simulink library "tqr"  (R2021b)
settings: Solver=VariableStepAuto  StartTime=0.0  StopTime=10.0  RelTol=1e-3
undefined symbols (not defined in the file or in its folder): ATQR_AltRDCActiveFEDUInc_X_pct, ATQR_AltRDCActiveFEDUInc_Y_enum, ATQR_AltRDCActiveFEDUTs_X_pct, ATQR_AltRDCActiveFEDUTs_Y_enum, ATQR_AltRDCActiveREDUInc_X_pct, ATQR_AltRDCActiveREDUInc_Y_enum, ATQR_AltRDCActiveREDUTs_X_pct, ATQR_AltRDCActiveREDUTs_Y_enum, ATQR_CreepFEDUTqIncSR_X_rpm, ATQR_CreepFEDUTqIncSR_Y_Nm, ATQR_CreepFEDUTs_X_rpm, ATQR_CreepFEDUTs_Y_Nm, ATQR_EcoTqFrIncGain_X_Nm, ATQR_EcoTqFrIncGain_Y_pct, ATQR_EcoTqRrIncGain_X_Nm, ATQR_EcoTqRrIncGain_Y_pct, ATQR_EL1FEDUTqDecSR_Y_Nm, ATQR_EL1FEDUTqIncSR_X_rpm, ATQR_EL1FEDUTqIncSR_Y_pct, ATQR_EL1FEDUTs_X_rpm, ATQR_EL1FEDUTs_Y_Nm, ATQR_EL1REDUTqDecSR_Y_Nm, ATQR_EL1REDUTs_Y_Nm, ATQR_FEDUEL1RegenTs_X_rpm, ATQR_FEDUTIPOutTs_X_rpm, ATQR_FrNegRateLimitIncN_X_rpm, ATQR_FrNegRateLimitIncN_Y_Nm, ATQR_FrPosRateLimitIncN_X_rpm, ATQR_FrPosRateLimitIncN_Y_Nm, ATQR_FShaftSpdTqLimCoe_X_rpm, ATQR_FTimerTqLimCoe_X_s, ATQR_FTqZeroTransUpBoundN_X_rpm, ATQR_NL1FEDUTqDecSR_Y_Nm, ATQR_NL1FEDUTqIncSR_X_rpm, ATQR_NL1FEDUTqIncSR_Y_pct, ATQR_NL1FEDUTs_X_rpm, ATQR_NL1FEDUTs_Y_Nm, ATQR_NL1REDUTqDecSR_Y_Nm, ATQR_NL1REDUTs_Y_Nm, ATQR_NormalTqFrIncGain_X_Nm, ATQR_NormalTqFrIncGain_Y_pct, ATQR_NormalTqRrIncGain_X_Nm, ATQR_NormalTqRrIncGain_Y_pct, ATQR_RrNegRateLimitIncN_X_rpm, ATQR_RrNegRateLimitIncN_Y_Nm, ATQR_RrPosRateLimitIncN_X_rpm, ATQR_RrPosRateLimitIncN_Y_Nm, ATQR_RShaftSpdTqLimCoe_X_rpm, ATQR_RTimerTqLimCoe_X_s, ATQR_SL1FEDUTqDecSR_Y_Nm, ATQR_SL1FEDUTqIncSR_X_rpm, ATQR_SL1FEDUTqIncSR_Y_pct, ATQR_SL1FEDUTs_X_rpm, ATQR_SL1FEDUTs_Y_Nm, ATQR_SL1REDUTqDecSR_Y_Nm, ATQR_SL1REDUTs_Y_Nm, ATQR_SportTqFrIncGain_X_Nm, ATQR_SportTqFrIncGain_Y_pct, ATQR_SportTqRrIncGain_X_Nm, ATQR_SportTqRrIncGain_Y_pct ... (+287)
libraries: hcu_lib x19, simulink x17, $bdroot x3
(part 2 of 10)

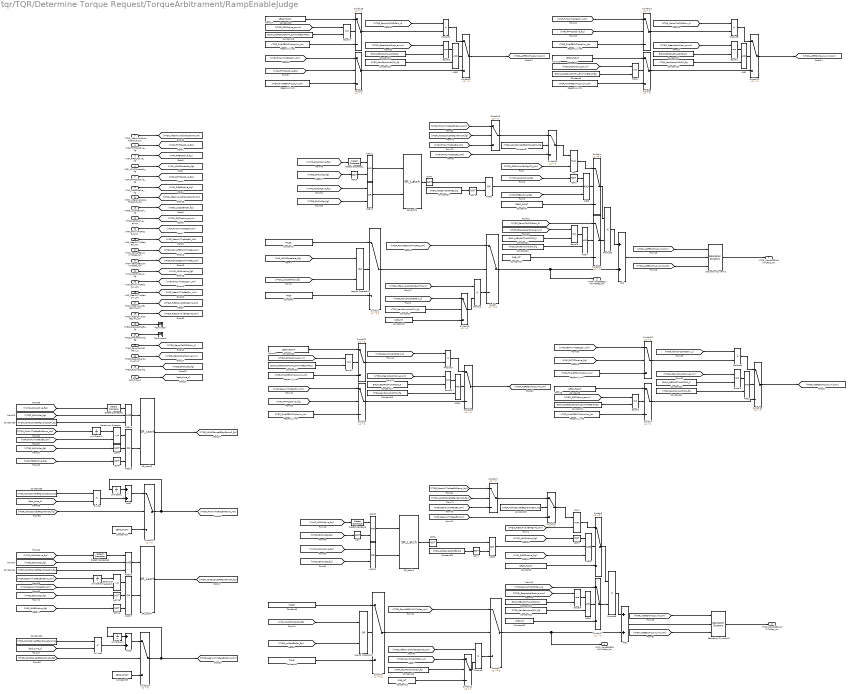
== system tqr/TQR/Determine Torque Request/TorqueArbitrament/RampEnableJudge ==
  VTQD_AfterAvailableTqDemFr_Nm : Inport
  VINP_FrPTCSActive_flg : Inport  Port=2
  VINP_FrRBCActive_flg : Inport  Port=3
  VINP_ADASForceIdle_flg : Inport  Port=4
  VTQR_RampFEDUWhlTqReq_Nm : Inport  Port=5
  VTQD_AfterAvailableTqDemRr_Nm : Inport  Port=6
  VINP_RrPTCSActive_flg : Inport  Port=7
  VINP_RrRBCActive_flg : Inport  Port=8
  VTQR_RampREDUWhlTqReq_Nm : Inport  Port=9
  VTQD_LoSpdBrkCtrl_flg : Inport  Port=10
  VTQD_RDCActive_enum : Inport  Port=11
  VINP_FrntAxlTrqReqBrk_Nm : Inport  Port=12
  VINP_RearAxlTrqReqBrk_Nm : Inport  Port=13
  VVMC_ADASActive_flg : Inport  Port=14
  VINP_FrntAxlTrqReqDrv_Nm : Inport  Port=15
  VINP_RearAxlTrqReqDrv_Nm : Inport  Port=16
  VTQD_FrEDUAvailBrkRgnTq_Nm : Inport  Port=17
  VTQD_RrEDUAvailBrkRgnTq_Nm : Inport  Port=18
  VTQD_PreLoadPreEn_flg : Inport  Port=19
  VTQD_PreLoadHold_flg : Inport  Port=20
  VTQR_RampTqCMDGain_c : Inport  Port=21
  VTQD_GearActualPosn_enum : Inport  Port=22
  VTQD_BrkSwSta_flg : Inport  Port=23
  task_time_s : Inport  Port=24
  AND{,1..2,4,6..7,10,12} (8 alike) : Logic  AllPortsSameDT=off  OutDataTypeStr=boolean
  AND{8..9,11,13} (4 alike) : Logic  Operator=OR  AllPortsSameDT=off  OutDataTypeStr=boolean
  AND{3,5,14,16} (4 alike) : Logic  Inputs=3  AllPortsSameDT=off  OutDataTypeStr=boolean
  AND15 : Logic  Operator=OR  Inputs=3  AllPortsSameDT=off  OutDataTypeStr=boolean
  AND17 : Logic  Operator=OR  Inputs=3  AllPortsSameDT=off  OutDataTypeStr=boolean
  Add{,1..3} (4 alike) : Sum
  Constant : Constant  Value=TRUE
  Constant1 : Constant  Value=FALSE
  Constant{10,12,14,22} (4 alike) : Constant  Value=ONE_INT
  Constant{6,11,18,28} (4 alike) : Constant  Value=ENUM_CANRDCACTSTA_EXITIMMEDIATELY
  Constant{9,13,15..16,20,24,26,30} (8 alike) : Constant  Value=KTQR_NewRampArchSW_flg
  Constant{17,21,23,25,27,31} (6 alike) : Constant  Value=ENUM_GEARACTUALPOSN_R
  Constant{4..5,7..8,19,29,34,39} (8 alike) : Constant  Value=ZERO_FLOAT
  Constant2 : Constant  Value=TRUE
  Constant3 : Constant  Value=FALSE
  Constant32 : Constant  Value=KTQR_ACCCancelNoRBC_flg
  Constant33 : Constant  Value=KTQR_ACCCancelNoRBC_flg
  Constant35 : Constant  Value=KTQR_ADASCancelBRgnSlopeF_Nmps
  Constant{36..38,41} (4 alike) : Constant  Value=KTQR_ADASCancelBRgnSlopeSW_flg
  Constant40 : Constant  Value=KTQR_ADASCancelBRgnSlopeR_Nmps
  Detect Decrease{,1..3} (4 alike) : simulink/Logic and Bit Operations/Detect Decrease  vinit=0.0  OutDataTypeStr=boolean
  Divide : Product  Inputs=**
  Divide1 : Product  Inputs=**
  Equal{,1..9} (10 alike) : RelationalOperator  Operator===  OutDataTypeStr=boolean  RndMeth=Simplest
  Logical Operator1 : Logic  Operator=OR  AllPortsSameDT=off  OutDataTypeStr=boolean
  Logical Operator2 : Logic  Operator=OR  AllPortsSameDT=off  OutDataTypeStr=boolean
  Max : MinMax  Function=max  Inputs=2
  Max1 : MinMax  Function=max  Inputs=2
  NOT{,1..11} (12 alike) : Logic  Operator=NOT  AllPortsSameDT=off  OutDataTypeStr=boolean
  Product{,1..7} (8 alike) : Product
  RegenLV_inc1 : Constant  Value=KTQR_FinalFEDUTrqLowLim_Nm  OutDataTypeStr=single
  RegenLV_inc2 : Constant  Value=KTQR_FinalFEDUTrqUpLim_Nm  OutDataTypeStr=single
  RegenLV_inc3 : Constant  Value=KTQR_FinalREDUTrqLowLim_Nm  OutDataTypeStr=single
  RegenLV_inc4 : Constant  Value=KTQR_FinalREDUTrqUpLim_Nm  OutDataTypeStr=single
  RegenLV_inc5 : Constant  Value=KTQR_FinalFEDUTrqUpLim_Nm  OutDataTypeStr=single
  RegenLV_inc6 : Constant  Value=KTQR_FinalFEDUTrqLowLim_Nm  OutDataTypeStr=single
  RegenLV_inc7 : Constant  Value=KTQR_FinalREDUTrqUpLim_Nm  OutDataTypeStr=single
  RegenLV_inc8 : Constant  Value=KTQR_FinalREDUTrqLowLim_Nm  OutDataTypeStr=single
  Relational Operator : RelationalOperator  Operator=<=  OutDataTypeStr=boolean  RndMeth=Simplest
  Relational Operator1 : RelationalOperator  Operator=<=  OutDataTypeStr=boolean  RndMeth=Simplest
  SR_Latch{1..4} (4 alike) : hcu_lib/Basic_Blocks/SR_Latch
  Saturation Dynamic : simulink/Discontinuities/Saturation Dynamic  OutMin=[]  OutMax=[]  OutDataTypeStr=Inherit: Same as second input  OutDataType=fixdt(1, 16)  OutScaling=2^-10  DoSatur=off
  Saturation Dynamic1 : simulink/Discontinuities/Saturation Dynamic  OutMin=[]  OutMax=[]  OutDataTypeStr=Inherit: Same as second input  OutDataType=fixdt(1, 16)  OutScaling=2^-10  DoSatur=off
  Switch{,1..5} (6 alike) : Switch  Criteria=u2 ~= 0
  Switch{6..27} (22 alike) : Switch  Criteria=u2 > Threshold
  Terminator : Terminator
  Terminator1 : Terminator
  Unit Delay{,1..3} (4 alike) : UnitDelay  SampleTime=-1  HasFrameUpgradeWarning=on
  VTQR_ActualFEDUWhlTqReq_Nm : Outport
  VTQR_ActualREDUWhlTqReq_Nm : Outport  Port=2
  VTQR_NoABSFEDUWhlTqReq_Nm : Outport  Port=3
  VTQR_NoABSREDUWhlTqReq_Nm : Outport  Port=4
  wires:
  VINP_ADASForceIdle_flg/1 -> [VINP_ADASForceIdle_flg]
  VINP_FrPTCSActive_flg/1 -> [VINP_FrPTCSActive_flg]
  VINP_RrPTCSActive_flg/1 -> [VINP_RrPTCSActive_flg]
  VINP_FrRBCActive_flg/1 -> [VINP_FrRBCActive_flg]
  VINP_RrRBCActive_flg/1 -> [VINP_RrRBCActive_flg]
  VTQD_LoSpdBrkCtrl_flg/1 -> [VTQD_LoSpdBrkCtrl_flg]
  VTQD_RDCActive_enum/1 -> [VTQD_RDCActive_enum]
  VINP_FrntAxlTrqReqBrk_Nm/1 -> [VINP_FrntAxlTrqReqBrk_Nm]
  VINP_RearAxlTrqReqBrk_Nm/1 -> [VINP_RearAxlTrqReqBrk_Nm]
  VTQR_RampFEDUWhlTqReq_Nm/1 -> [VTQR_RampFEDUWhlTqReq_Nm]
  VTQR_RampREDUWhlTqReq_Nm/1 -> [VTQR_RampREDUWhlTqReq_Nm]
  VVMC_ADASActive_flg/1 -> [VVMC_ADASActive_flg]
  VTQD_AfterAvailableTqDemFr_Nm/1 -> [VTQD_AfterAvailableTqDemFr_Nm]
  VTQD_AfterAvailableTqDemRr_Nm/1 -> [VTQD_AfterAvailableTqDemRr_Nm]
  VINP_RearAxlTrqReqDrv_Nm/1 -> [VINP_RearAxlTrqReqDrv_Nm]
  VINP_FrntAxlTrqReqDrv_Nm/1 -> [VINP_FrntAxlTrqReqDrv_Nm]
  Constant7/1 -> Switch6/1
  [VINP_ADASForceIdle_flg] -> Logical Operator1/1
  [VINP_FrPTCSActive_flg] -> Switch8/2
  Constant2/1 -> Switch3/3
  Constant6/1 -> Equal/2
  RegenLV_inc2/1 -> Switch8/3
  Constant1/1 -> Switch2/1
  [VTQR_RampREDUWhlTqReq_Nm] -> Switch1/1
  Switch2/1 -> Switch/2  "VTQR_FrRampEnable_flg"
  Constant3/1 -> Switch3/1
  Saturation Dynamic/1 -> VTQR_ActualFEDUWhlTqReq_Nm/1  "VTQR_ActualFEDUWhlTqReq_Nm"
  Logical Operator1/1 -> Switch2/2
  RegenLV_inc4/1 -> Switch9/3
  Constant8/1 -> Switch7/1
  Equal4/1 -> Switch7/2
  Constant11/1 -> Equal4/2
  [VTQD_RDCActive_enum] -> Equal/1
  [VINP_FrntAxlTrqReqDrv_Nm] -> Switch8/1
  Constant5/1 -> Switch5/3
  Equal/1 -> Switch6/2
  Switch3/1 -> Switch1/2  "VTQR_RrRampEnable_flg"
  [VTQD_RDCActive_enum] -> Equal4/1
  NOT1/1 -> AND3/1
  Logical Operator2/1 -> Switch3/2
  Add1/1 -> Saturation Dynamic1/2
  [VINP_RearAxlTrqReqDrv_Nm] -> Switch9/1
  Saturation Dynamic1/1 -> VTQR_ActualREDUWhlTqReq_Nm/1  "VTQR_ActualREDUWhlTqReq_Nm"
  [VTQR_RampFEDUWhlTqReq_Nm] -> Switch/1
  Add/1 -> Saturation Dynamic/2
  Constant/1 -> Switch2/3
  [VVMC_ADASActive_flg] -> NOT2/1
  NOT2/1 -> AND5/1
  AND3/1 -> Switch4/2
  AND5/1 -> Switch5/2
  [VVMC_ADASActive_flg] -> NOT1/1
  [VINP_RrRBCActive_flg] -> AND5/3
  Switch/1 -> VTQR_NoABSFEDUWhlTqReq_Nm/1, Add/2  "VTQR_NoABSFEDUWhlTqReq_Nm"
  Constant4/1 -> Switch4/3
  Switch1/1 -> Add1/2, VTQR_NoABSREDUWhlTqReq_Nm/1  "VTQR_NoABSREDUWhlTqReq_Nm"
  RegenLV_inc1/1 -> Switch6/3
  [VINP_RrPTCSActive_flg] -> Switch9/2
  [VINP_FrRBCActive_flg] -> AND3/3
  RegenLV_inc3/1 -> Switch7/3
  VTQD_FrEDUAvailBrkRgnTq_Nm/1 -> [VTQD_FrEDUAvailBrkRgnTq_Nm]
  VTQD_RrEDUAvailBrkRgnTq_Nm/1 -> [VTQD_RrEDUAvailBrkRgnTq_Nm]
  Max/1 -> Switch4/1
  [VTQD_FrEDUAvailBrkRgnTq_Nm] -> Max/2
  Max1/1 -> Switch5/1
  [VTQD_RrEDUAvailBrkRgnTq_Nm] -> Max1/2
  VTQD_PreLoadHold_flg/1 -> Terminator1/1
  VTQD_PreLoadPreEn_flg/1 -> Terminator/1
  [VINP_ADASForceIdle_flg] -> Logical Operator2/1
  [VTQD_LoSpdBrkCtrl_flg] -> Logical Operator1/2
  [VTQD_LoSpdBrkCtrl_flg] -> Logical Operator2/2
  VTQR_RampTqCMDGain_c/1 -> [VTQR_RampTqCMDGain_c]
  Product/1 -> Switch/3
  [VTQD_AfterAvailableTqDemFr_Nm] -> Product/1
  Switch10/1 -> Product/2
  [VTQR_RampTqCMDGain_c] -> Switch10/1
  Constant9/1 -> Switch10/2
  Constant10/1 -> Switch10/3
  Constant13/1 -> Switch11/2
  Switch11/1 -> Product1/2
  Constant12/1 -> Switch11/3
  Product1/1 -> Switch1/3
  [VTQD_AfterAvailableTqDemRr_Nm] -> Product1/1
  [VTQR_RampTqCMDGain_c] -> Switch11/1
  Constant14/1 -> Switch12/3
  [VTQR_RampTqCMDGain_c] -> Switch12/1
  Switch12/1 -> Product2/2
  Product2/1 -> Add/1
  Switch4/1 -> Product2/1
  [VTQR_ActFEDUTqLowLimit_Nm] -> Saturation Dynamic/3
  Switch6/1 -> Switch13/3
  Switch13/1 -> [VTQR_ActFEDUTqLowLimit_Nm]  "VTQR_ActFEDUTqLowLimit_Nm"
  AND/1 -> Switch13/2
  Constant16/1 -> AND/2
  VTQD_GearActualPosn_enum/1 -> [VTQD_GearActualPosn_enum]
  Equal1/1 -> AND/1
  [VTQD_GearActualPosn_enum] -> Equal1/1
  Constant17/1 -> Equal1/2
  [VINP_FrPTCSActive_flg] -> Switch14/2
  [VINP_FrntAxlTrqReqDrv_Nm] -> Switch14/1
  RegenLV_inc5/1 -> Switch14/3
  Product3/1 -> Switch13/1
  Switch14/1 -> Product3/2
  [VTQR_RampTqCMDGain_c] -> Product3/1
  Equal2/1 -> Switch15/2
  RegenLV_inc6/1 -> Switch15/3
  [VTQD_RDCActive_enum] -> Equal2/1
  Constant18/1 -> Equal2/2
  Constant19/1 -> Switch15/1
  [VTQR_RampTqCMDGain_c] -> Product4/1
  AND1/1 -> Switch16/2
  Equal3/1 -> AND1/1
  Constant21/1 -> Equal3/2
  Product4/1 -> Switch16/1
  Constant20/1 -> AND1/2
  [VTQD_GearActualPosn_enum] -> Equal3/1
  Switch15/1 -> Product4/2
  Switch8/1 -> Switch16/3
  Switch16/1 -> [VTQR_ActFEDUTqUpLimit_Nm]  "VTQR_ActFEDUTqUpLimit_Nm"
  [VTQR_RampTqCMDGain_c] -> Switch17/1
  Constant22/1 -> Switch17/3
  Switch5/1 -> Product5/1
  Product5/1 -> Add1/1
  [VTQR_ActREDUTqLowLimit_Nm] -> Saturation Dynamic1/3
  [VTQR_RampTqCMDGain_c] -> Product6/1
  AND2/1 -> Switch18/2
  Equal5/1 -> AND2/1
  Constant25/1 -> Equal5/2
  Product6/1 -> Switch18/1
  Constant24/1 -> AND2/2
  [VTQD_GearActualPosn_enum] -> Equal5/1
  Switch19/1 -> Product6/2
  Switch7/1 -> Switch18/3
  Switch18/1 -> [VTQR_ActREDUTqLowLimit_Nm]  "VTQR_ActREDUTqLowLimit_Nm"
  [VINP_RrPTCSActive_flg] -> Switch19/2
  [VINP_RearAxlTrqReqDrv_Nm] -> Switch19/1
  RegenLV_inc7/1 -> Switch19/3
  Product7/1 -> Switch20/1
  Constant27/1 -> Equal6/2
  [VTQD_GearActualPosn_enum] -> Equal6/1
  Equal6/1 -> AND4/1
  Constant26/1 -> AND4/2
  [VTQR_RampTqCMDGain_c] -> Product7/1
  Switch21/1 -> Product7/2
  AND4/1 -> Switch20/2
  Switch9/1 -> Switch20/3
  Switch20/1 -> [VTQR_ActREDUTqUpLimit_Nm]  "VTQR_ActREDUTqUpLimit_Nm"
  [VTQR_ActREDUTqUpLimit_Nm] -> Saturation Dynamic1/1
  [VTQR_ActFEDUTqUpLimit_Nm] -> Saturation Dynamic/1
  RegenLV_inc8/1 -> Switch21/3
  Constant29/1 -> Switch21/1
  Equal7/1 -> Switch21/2
  Constant28/1 -> Equal7/2
  [VTQD_RDCActive_enum] -> Equal7/1
  Switch17/1 -> Product5/2
  Equal8/1 -> AND6/1
  Constant23/1 -> Equal8/2
  Constant15/1 -> AND6/2
  [VTQD_GearActualPosn_enum] -> Equal8/1
  AND6/1 -> Switch17/2
  Constant30/1 -> AND7/2
  [VTQD_GearActualPosn_enum] -> Equal9/1
  Constant31/1 -> Equal9/2
  Equal9/1 -> AND7/1
  AND7/1 -> Switch12/2
  NOT3/1 -> AND8/2
  Constant32/1 -> NOT3/1
  AND8/1 -> AND3/2
  Constant33/1 -> NOT4/1
  NOT4/1 -> AND9/2
  AND9/1 -> AND5/2
  VTQD_BrkSwSta_flg/1 -> [VTQD_BrkSwSta_flg]
  [VVMC_ADASActive_flg] -> Detect Decrease/1
  [VTQD_BrkSwSta_flg] -> NOT/1
  AND10/1 -> SR_Latch1/1
  Detect Decrease/1 -> AND10/1
  [VVMC_ADASActive_flg] -> AND11/1
  NOT/1 -> AND10/2
  [VTQD_BrkSwSta_flg] -> AND11/2
  AND11/1 -> SR_Latch1/2
  SR_Latch1/1 -> NOT6/1
  [VTQD_BrkSwSta_flg] -> AND13/2
  [VTQD_BrkSwSta_flg] -> NOT5/1
  AND13/1 -> SR_Latch2/2
  NOT5/1 -> AND12/2
  Detect Decrease1/1 -> AND12/1
  [VVMC_ADASActive_flg] -> Detect Decrease1/1
  AND12/1 -> SR_Latch2/1
  [VVMC_ADASActive_flg] -> AND13/1
  SR_Latch2/1 -> NOT7/1
  NOT6/1 -> AND9/1
  NOT7/1 -> AND8/1
  [VTQR_FrntAxlTrqReqBrkRamp_Nm] -> Switch26/1
  [VINP_FrntAxlTrqReqBrk_Nm] -> Switch23/3
  [VTQR_ADASCancelBRgnRampF_flg] -> Switch26/2
  [VINP_FrntAxlTrqReqBrk_Nm] -> Switch26/3
  Switch26/1 -> Switch23/1
  Constant37/1 -> Switch23/2
  Switch23/1 -> Max/1
  NOT10/1 -> AND17/2
  Divide/1 -> Add2/2
  AND17/1 -> SR_Latch4/2
  [VINP_RrRBCActive_flg] -> NOT11/1
  [VTQD_BrkSwSta_flg] -> AND14/2
  AND16/1 -> SR_Latch4/1
  Add3/1 -> Switch25/1
  Unit Delay3/1 -> Relational Operator1/1
  Switch25/1 -> Unit Delay1/1, [VTQR_RearAxlTrqReqBrkRamp_Nm]  "VTQR_RearAxlTrqReqBrkRamp_Nm"
  Detect Decrease3/1 -> AND16/1
  Relational Operator1/1 -> AND17/1
  [VTQD_BrkSwSta_flg] -> NOT10/1
  [VTQR_ADASCancelBRgnRampR_flg] -> Switch25/2
  Divide1/1 -> Add3/2
  Constant41/1 -> AND16/3
  [VVMC_ADASActive_flg] -> Detect Decrease3/1
  [VTQD_BrkSwSta_flg] -> AND16/2
  [VINP_FrRBCActive_flg] -> NOT9/1
  [VTQD_BrkSwSta_flg] -> NOT8/1
  Constant39/1 -> Switch25/3
  [VTQR_RearAxlTrqReqBrkRamp_Nm] -> Unit Delay3/1
  NOT9/1 -> AND15/3
  [task_time_s] -> Divide/2
  Switch22/1 -> Unit Delay/1, [VTQR_FrntAxlTrqReqBrkRamp_Nm]  "VTQR_FrntAxlTrqReqBrkRamp_Nm"
  NOT8/1 -> AND15/2
  [VVMC_ADASActive_flg] -> Detect Decrease2/1
  NOT11/1 -> AND17/3
  Detect Decrease2/1 -> AND14/1
  Constant34/1 -> Switch22/3
  Constant36/1 -> AND14/3
  [VTQR_ADASCancelBRgnRampF_flg] -> Switch22/2
  Unit Delay/1 -> Add2/1
  [VINP_RearAxlTrqReqBrk_Nm] -> Relational Operator1/2
  Constant40/1 -> Divide1/1
  AND14/1 -> SR_Latch3/1
  [task_time_s] -> Divide1/2
  SR_Latch4/1 -> [VTQR_ADASCancelBRgnRampR_flg]  "VTQR_ADASCancelBRgnRampR_flg"
  Constant35/1 -> Divide/1
  SR_Latch3/1 -> [VTQR_ADASCancelBRgnRampF_flg]  "VTQR_ADASCancelBRgnRampF_flg"
  Unit Delay1/1 -> Add3/1
  Relational Operator/1 -> AND15/1
  AND15/1 -> SR_Latch3/2
  Add2/1 -> Switch22/1
  [VTQR_FrntAxlTrqReqBrkRamp_Nm] -> Unit Delay2/1
  [VINP_FrntAxlTrqReqBrk_Nm] -> Relational Operator/2
  Unit Delay2/1 -> Relational Operator/1
  Switch24/1 -> Max1/1
  [VTQR_RearAxlTrqReqBrkRamp_Nm] -> Switch27/1
  Switch27/1 -> Switch24/1
  [VTQR_ADASCancelBRgnRampR_flg] -> Switch27/2
  [VINP_RearAxlTrqReqBrk_Nm] -> Switch24/3
  [VINP_RearAxlTrqReqBrk_Nm] -> Switch27/3
  Constant38/1 -> Switch24/2
  task_time_s/1 -> [task_time_s]

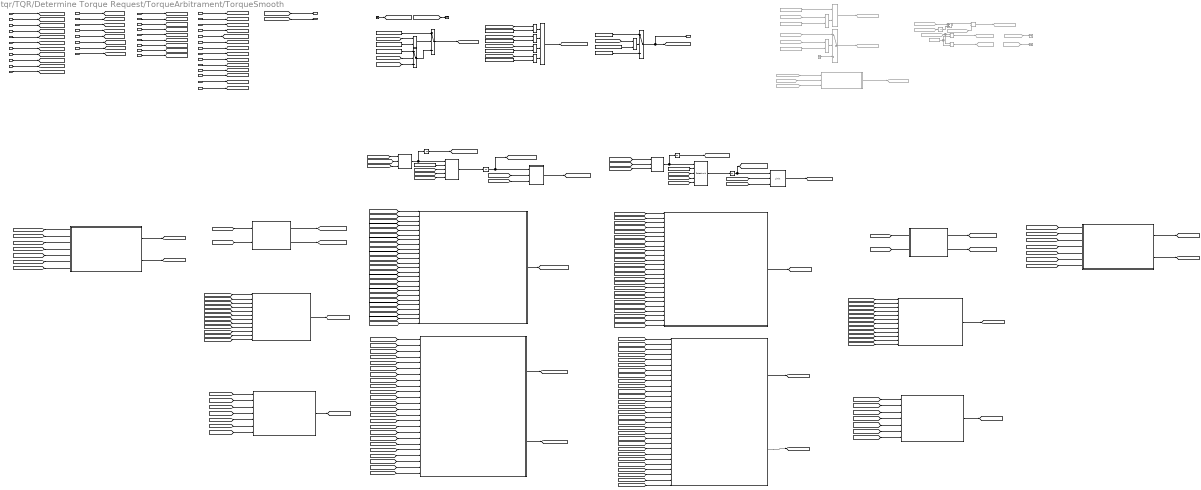
== system tqr/TQR/Determine Torque Request/TorqueArbitrament/TorqueSmooth ==
  note: Fr | Rr
  note: Front First order filter input tau map and determination
  note: Rear Rate limitation map and determination
  note: Front Rate limitation map and determination
  note: Rear wheel first order filter input torque command determination
  note: Front wheel first order filter input torque command determination:
  note: Rear Torque zero point transfer status determination
  note: Front Torque zero point transfer status determination
  note: Front Torque zero point transfer boundary map
  note: Rear Torque zero point transfer boundary map
  note: Rear First order filter input tau map and determination
  note: Rear torque ramp limtation and determination
  note: Rear torque ramp limtation and determination
  note: Rear Final Torque
  note: Front Final Torque
  task_time_s : Inport
  VDHP_ActAPSPosn_pct : Inport  Port=2
  VTQD_TqTargetShaftSpd_rpm : Inport  Port=3
  VTQD_TqSourceFr_enum : Inport  Port=4
  VTQD_TqSourceRr_enum : Inport  Port=5
  VTQD_AfterAvailableTqDemRr_Nm : Inport  Port=6
  VTQD_AfterAvailableTqDemFr_Nm : Inport  Port=7
  VTQD_EVDriveMode_enum : Inport  Port=8
  VTQD_EVDriveModeValid_flg : Inport  Port=9
  VTQD_RollRegenEnable_flg : Inport  Port=10
  VINP_VehSpeed_kph : Inport  Port=11
  VPMM_DriveTrainSelect_enum : Inport  Port=12
  VTQD_LimpHomeAct_flg : Inport  Port=13
  VTQD_RegenMode_enum : Inport  Port=14
  VVMC_ACCPedalOvrd_flg : Inport  Port=15
  VVMC_CCPedalOvrd_flg : Inport  Port=16
  VTQD_GearActualPosn_enum : Inport  Port=17
  VTQD_PreLoadHold_flg : Inport  Port=18
  VTQD_PreLoadPreEn_flg : Inport  Port=19
  VTQR_NoABSFEDUWhlTqReq_Nm : Inport  Port=20
  VTQR_NoABSREDUWhlTqReq_Nm : Inport  Port=21
  VTQD_CreepPrLoadEnable_flg : Inport  Port=22
  VVMC_ADASActive_flg : Inport  Port=23
  VTQD_RDCActive_enum : Inport  Port=24
  VVMC_ActMaxSlideRate_pct : Inport  Port=25
  VTQD_RegenTqLimitEn_flg : Inport  Port=26
  VTQD_PedAccTqEn_flg : Inport  Port=27
  VTQR_FrGearChange_flg : Inport  Port=28
  VTQR_RrGearChange_flg : Inport  Port=29
  VVMC_MSAWhlTqActive_flg : Inport  Port=30
  VINP_LFRawWhlSpeed_kph : Inport  Port=31
  VINP_RFRawWhlSpeed_kph : Inport  Port=32
  VINP_LRRawWhlSpeed_kph : Inport  Port=33
  VINP_RRRawWhlSpeed_kph : Inport  Port=34
  VINP_ACCVehHoldReq_flg : Inport  Port=35
  VINP_GRADE_Deg : Inport  Port=36
  VTQD_VehActSpd_kph : Inport  Port=37
  VVMC_EstSlope_Deg : Inport  Port=38
  VINP_RrPTCSActive_flg : Inport  Port=39
  VINP_FrPTCSActive_flg : Inport  Port=40
  VINP_IVISnowModeCmd_flg : Inport  Port=41
  VINP_VehicleType_enum : Inport  Port=42
  AND : Logic  Inputs=4  AllPortsSameDT=off  OutDataTypeStr=boolean
  AND18 : Logic  Commented=on  AllPortsSameDT=off  OutDataTypeStr=boolean
  Constant : Constant  Value=ZERO_FLOAT
  Constant1 : Constant  Value=ZERO_FLOAT
  Constant2 : Constant  Value=ENUM_REGENLEVEL_LV1
  Constant3 : Constant  Value=MINUSONE_FLOAT
  Constant36 : Constant  Commented=on  Value=KTQR_AWDSynchEnbl_flg
  Constant38 : Constant  Commented=on  Value=ENUM_DRIVETRAIN_AWD
  Constant4 : Constant  Value=ENUM_DRIVEMODE_SPORT
  Constant41 : Constant  Commented=on  Value=ZERO_INT
  Constant47 : Constant  Commented=on  Value=ENUM_DRIVETRAIN_FWD
  Constant5 : Constant  Value=KTQR_LaunchEnPedal_pct
  Constant6 : Constant  Value=KTQR_LaunchEnSpd_kph
  Constant7 : Constant  Value=ONE_FLOAT
  Divide : Product  Commented=on  Inputs=*/
  Equal{,1..3} (4 alike) : RelationalOperator  Operator===  OutDataTypeStr=boolean  RndMeth=Simplest
  Equal34 : RelationalOperator  Commented=on  Operator===  OutDataTypeStr=boolean  RndMeth=Simplest
  Equal35 : RelationalOperator  Commented=on  Operator===  OutDataTypeStr=boolean  RndMeth=Simplest
  FirstOrderFilter : Subsystem  RTWFileName=HCU_LIB  mask(FirstOrderFilter){}
      mask help: First order Filter.
      settings: RTWFileNameOpts=User specified
  FirstOrderFilter1 : $bdroot/TQR/Determine Torque Request/TorqueArbitrament/TorqueSmooth/FirstOrderFilter
  From125 : From  Commented=on  GotoTag=VDHP_ActAPSPosn_pct
  From127 : From  Commented=on  GotoTag=VTQR_ActAPSPosnAcc_enum
  From139 : From  Commented=on  GotoTag=VTQR_PedalAcc_flg
  From140 : From  Commented=on  GotoTag=VTQR_PedalDec_flg
  From141 : From  Commented=on  GotoTag=VDHP_ActAPSPosn_pct
  From142 : From  Commented=on  GotoTag=task_time_s
  From153 : From  Commented=on  GotoTag=VTQD_TqTargetShaftSpd_rpm
  From154 : From  Commented=on  GotoTag=VPMM_DriveTrainSelect_enum
  From155 : From  Commented=on  GotoTag=VPMM_DriveTrainSelect_enum
  From5 : From  Commented=on  GotoTag=VTQD_DRTransfer_flg
      settings: CloseFcn=tagdialog Close
  From6 : From  Commented=on  GotoTag=NTQR_TMTqReq_Nm
      settings: CloseFcn=tagdialog Close
  From9 : From  Commented=on  GotoTag=VTQR_TMTqReqLimit_Nm
      settings: CloseFcn=tagdialog Close
  Front First order filter input tau map and determination : Subsystem
  Front Torque zero point transfer boundary map : Subsystem
  "Front Torque zero point transfer status determination " : Subsystem
  Front torque ramp limtation and determination : Subsystem
  Front wheel first order filter input torque command determination : Subsystem
  Front wheel rate limit determination : Subsystem
  Goto19 : Goto  Commented=on  GotoTag=VTQR_AWDSynchEnbl_flg
  Goto2 : Goto  Commented=on  GotoTag=VTQR_ZeroTqRecover_flg
  Goto22 : Goto  Commented=on  GotoTag=VTQR_ActAPSPosnAcc_enum
  Goto23 : Goto  Commented=on  GotoTag=VTQR_PedalAcc_flg
  Goto24 : Goto  Commented=on  GotoTag=VTQR_PedalDec_flg
  Goto9 : Goto  Commented=on  GotoTag=VTQD_CAN2TqTargetShaftSpd_rpm
  GreaterThan : RelationalOperator  Commented=on  Operator=>  OutDataTypeStr=boolean  RndMeth=Simplest
  Ground : Ground  Commented=on
  Ground1 : Ground
  Less Than : RelationalOperator  Commented=on  Operator=<  OutDataTypeStr=boolean  RndMeth=Simplest
  Limit : Subsystem  RTWFileName=HCU_LIB  mask(Limit){}
      mask help: Limit funcion.
      settings: RTWFileNameOpts=User specified
  Limit2 : $bdroot/TQR/Determine Torque Request/TorqueArbitrament/TorqueSmooth/Limit
  RateLimit : Subsystem  RTWFileName=HCU_LIB  mask(RateLimit){}
      mask help: Rate limit function.
      settings: RTWFileNameOpts=User specified
  RateLimit1 : $bdroot/TQR/Determine Torque Request/TorqueArbitrament/TorqueSmooth/RateLimit
  Rear First order filter input tau map and determination : Subsystem
  Rear Torque zero point transfer boundary map : Subsystem
  "Rear Torque zero point transfer status determination " : Subsystem
  Rear torque ramp limtation and determination : Subsystem
  Rear wheel first order filter input torque command determination : Subsystem
  Rear wheel rate limit determination : Subsystem
  RegenLV_inc1 : Constant  Value=ENUM_GEARACTUALPOSN_R
  RegenLV_inc2 : Constant  Value=ENUM_DRIVEMODE_ECO
  RegenLV_inc5 : Constant  Value=ENUM_GEARACTUALPOSN_R
  RegenLV_inc6 : Constant  Value=ENUM_DRIVEMODE_NRM
  Relational Operator4 : RelationalOperator  Operator=>  OutDataTypeStr=boolean  RndMeth=Simplest
  Relational Operator6 : RelationalOperator  Operator=<=  OutDataTypeStr=boolean  RndMeth=Simplest
  Subtract : Sum  Commented=on  Inputs=+-
  Switch : Switch  Criteria=u2 ~= 0
  Switch1 : Switch  Criteria=u2 > Threshold
  Switch10 : Switch  Commented=on  Criteria=u2 ~= 0
      settings: AttributesFormatString=<%<Criteria>>
  Switch2 : Switch  Criteria=u2 ~= 0
  Terminator : Terminator  Commented=on
  Terminator1 : Terminator  Commented=on
  Terminator2 : Terminator
  Unit Delay : UnitDelay  Commented=on  SampleTime=-1  HasFrameUpgradeWarning=on
  Unit Delay{1..4} (4 alike) : UnitDelay  SampleTime=-1
  Zero Torque Revert : Subsystem  Commented=on
  VTQR_RampFEDUWhlTqReq_Nm : Outport
  VTQR_RampREDUWhlTqReq_Nm : Outport  Port=2
  VTQR_RampTqCMDGain_c : Outport  Port=3
  wires:
  [task_time_s] -> FirstOrderFilter/2(Tc)
  FirstOrderFilter/1(out) -> Unit Delay3/1, RateLimit/1(input_raw)  "VTQR_FrFirstOrderOutTq_Nm"
  task_time_s/1 -> [task_time_s]
  RateLimit/1(output) -> Unit Delay1/1  "VTQR_FEDUWhlTqReqSmooth_Nm"
  Unit Delay1/1 -> [VTQR_FEDUWhlTqReqSmoothDelay_Nm], Limit/1(input)  "VTQR_FEDUWhlTqReqSmoothDelay_Nm"
  From5/1 -> Zero Torque Revert/1(VTQD_DRTransfer_flg)
  Zero Torque Revert/1(VTQR_ZeroTqRecover_flg) -> Goto2/1
  From6/1 -> Zero Torque Revert/2(NTQR_TMTqReq_Nm)
  From9/1 -> Zero Torque Revert/3(VTQR_TMTqReqLimit_Nm)
  [VTQR_ActFEDUTrqUpLim_Nm] -> Limit/2(upper_limit)
  [VTQR_ActFEDUTrqLowLim_Nm] -> Limit/3(lower_limit)
  Limit/1(out) -> [VTQR_RampFEDUWhlTqReq_Nm]  "VTQR_RampFEDUWhlTqReq_Nm"
  [task_time_s] -> RateLimit/3(steptime)
  Constant/1 -> RateLimit/2(initial_value)
  VTQD_TqSourceFr_enum/1 -> [VTQD_TqSourceFr_enum]
  VDHP_ActAPSPosn_pct/1 -> [VDHP_ActAPSPosn_pct]
  VTQD_AfterAvailableTqDemFr_Nm/1 -> [VTQD_AfterAvailableTqDemFr_Nm]
  VTQD_AfterAvailableTqDemRr_Nm/1 -> [VTQD_AfterAvailableTqDemRr_Nm]
  Unit Delay2/1 -> [VTQR_REDUWhlTqReqSmoothDelay_Nm], Limit2/1  "VTQR_REDUWhlTqReqSmoothDelay_Nm"
  RateLimit1/1 -> Unit Delay2/1  "VTQR_REDUWhlTqReqSmooth_Nm"
  FirstOrderFilter1/1 -> Unit Delay4/1, RateLimit1/1  "VTQR_RrFirstOrderOutTq_Nm"
  [task_time_s] -> FirstOrderFilter1/2
  Limit2/1 -> [VTQR_RampREDUWhlTqReq_Nm]  "VTQR_RampREDUWhlTqReq_Nm"
  [task_time_s] -> RateLimit1/3
  Constant1/1 -> RateLimit1/2
  VTQD_EVDriveMode_enum/1 -> [VTQD_EVDriveMode_enum]
  Constant38/1 -> Equal34/2
  Equal34/1 -> AND18/2
  From154/1 -> Equal34/1
  Constant36/1 -> AND18/1
  AND18/1 -> Goto19/1  "VTQR_AWDSynchEnbl_flg"
  From125/1 -> Subtract/1
  Divide/1 -> Goto22/1  "VTQR_ActAPSPosnAcc_enum"
  From127/1 -> Less Than/1, GreaterThan/1
  Constant41/1 -> Less Than/2, GreaterThan/2
  GreaterThan/1 -> Goto23/1  "VTQR_PedalAcc_flg"
  Less Than/1 -> Goto24/1  "VTQR_PedalDec_flg"
  From139/1 -> Terminator/1
  From140/1 -> Terminator1/1
  From141/1 -> Unit Delay/1
  Unit Delay/1 -> Subtract/2
  Subtract/1 -> Divide/1
  From142/1 -> Divide/2
  VTQD_RollRegenEnable_flg/1 -> [VTQD_RollRegenEnable_flg]
  VINP_VehSpeed_kph/1 -> [VINP_VehSpeed_kph]
  From155/1 -> Equal35/1
  Constant47/1 -> Equal35/2
  Equal35/1 -> Switch10/2
  Switch10/1 -> Goto9/1
  From153/1 -> Switch10/1
  VPMM_DriveTrainSelect_enum/1 -> [VPMM_DriveTrainSelect_enum]
  VTQD_LimpHomeAct_flg/1 -> [VTQD_LimpHomeAct_flg]
  VTQD_EVDriveModeValid_flg/1 -> [VTQD_EVDriveModeValid_flg]
  Ground/1 -> Switch10/3
  VTQD_TqSourceRr_enum/1 -> [VTQD_TqSourceRr_enum]
  Front wheel first order filter input torque command determination/1(VTQR_FrFirstOrderInpTq_Nm) -> [VTQR_FrFirstOrderInpTq_Nm]
  Rear wheel first order filter input torque command determination/1(VTQR_RrFirstOrderInpTq_Nm) -> [VTQR_RrFirstOrderInpTq_Nm]
  [VTQR_FrTqZeroTrans_enum] -> Front wheel rate limit determination/1(VTQR_FrTqZeroTrans_enum)
  [VTQD_TqSourceFr_enum] -> Front wheel rate limit determination/2(VTQD_TqSourceFr_enum)
  [VTQD_TqTargetShaftSpd_rpm] -> Front wheel rate limit determination/3(VTQD_TqTargetShaftSpd_rpm)
  Front wheel rate limit determination/2(VTQR_FrRateLimitDec_Nm) -> [VTQR_FrRateLimitDec_Nm]
  Front wheel rate limit determination/1(VTQR_FrRateLimitInc_Nm) -> [VTQR_FrRateLimitInc_Nm]
  [VTQR_FrFirstOrderInpTq_Nm] -> FirstOrderFilter/1(in)
  [VTQR_RrFirstOrderInpTq_Nm] -> FirstOrderFilter1/1
  [VTQR_FrRateLimitInc_Nm] -> RateLimit/4(ratelimt_inc)
  [VTQR_FrRateLimitDec_Nm] -> RateLimit/5(ratelimt_dec)
  Rear wheel rate limit determination/1(VTQR_RrRateLimitInc_Nm) -> [VTQR_RrRateLimitInc_Nm]
  Rear wheel rate limit determination/2(VTQR_RrRateLimitDec_Nm) -> [VTQR_RrRateLimitDec_Nm]
  [VTQD_TqTargetShaftSpd_rpm] -> Rear wheel rate limit determination/3(VTQD_TqTargetShaftSpd_rpm)
  [VTQD_TqSourceRr_enum] -> Rear wheel rate limit determination/2(VTQD_TqSourceRr_enum)
  [VTQR_RrTqZeroTrans_enum] -> Rear wheel rate limit determination/1(VTQR_RrTqZeroTrans_enum)
  [VTQR_RrRateLimitInc_Nm] -> RateLimit1/4
  [VTQR_RrRateLimitDec_Nm] -> RateLimit1/5
  Unit Delay3/1 -> [VTQR_FrFirstOrderOutTqDelay_Nm]  "VTQR_FrFirstOrderOutTqDelay_Nm"
  Front First order filter input tau map and determination/1(VTQR_FrFirstOrderInpTs_c) -> [VTQR_FrFirstOrderInpTs_c]
  [VTQR_FrFirstOrderInpTs_c] -> FirstOrderFilter/3(Ts)
  Rear First order filter input tau map and determination/1(VTQR_RrFirstOrderInpTs_c) -> [VTQR_RrFirstOrderInpTs_c]
  [VTQR_RrFirstOrderInpTs_c] -> FirstOrderFilter1/3
  Unit Delay4/1 -> [VTQR_RrFirstOrderOutTqDelay_Nm]  "VTQR_RrFirstOrderOutTqDelay_Nm"
  [VTQD_TqTargetShaftSpd_rpm] -> Front First order filter input tau map and determination/1(VTQD_TqTargetShaftSpd_rpm)
  [VTQR_EVDriveMode_enum] -> Front First order filter input tau map and determination/2(VTQR_EVDriveMode_enum)
  [VTQD_RollRegenEnable_flg] -> Front First order filter input tau map and determination/3(VTQD_RollRegenEnable_flg)
  [VTQD_TqSourceFr_enum] -> Front First order filter input tau map and determination/4(VTQD_TqSourceFr_enum)
  [VTQR_FEDUWhlTqReqSmoothDelay_Nm] -> Front First order filter input tau map and determination/5(VTQR_FEDUWhlTqReqSmoothDelay_Nm)
  [VDHP_ActAPSPosn_pct] -> Front First order filter input tau map and determination/6(VDHP_ActAPSPosn_pct)
  [VINP_VehSpeed_kph] -> Front First order filter input tau map and determination/7(VINP_VehSpeed_kph)
  [VTQD_LimpHomeAct_flg] -> Front First order filter input tau map and determination/8(VTQD_LimpHomeAct_flg)
  [VTQD_TqTargetShaftSpd_rpm] -> Rear First order filter input tau map and determination/1(VTQD_TqTargetShaftSpd_rpm)
  [VTQR_EVDriveMode_enum] -> Rear First order filter input tau map and determination/2(VTQR_EVDriveMode_enum)
  [VTQD_RollRegenEnable_flg] -> Rear First order filter input tau map and determination/3(VTQD_RollRegenEnable_flg)
  [VTQD_TqSourceRr_enum] -> Rear First order filter input tau map and determination/4(VTQD_TqSourceRr_enum)
  [VTQR_REDUWhlTqReqSmoothDelay_Nm] -> Rear First order filter input tau map and determination/5(VTQR_REDUWhlTqReqSmooth_Nm)
  [VDHP_ActAPSPosn_pct] -> Rear First order filter input tau map and determination/6(VDHP_ActAPSPosn_pct)
  [VINP_VehSpeed_kph] -> Rear First order filter input tau map and determination/7(VINP_VehSpeed_kph)
  [VTQD_LimpHomeAct_flg] -> Rear First order filter input tau map and determination/8(VTQD_LimpHomeAct_flg)
  [VTQD_LimpHomeAct_flg] -> Front wheel rate limit determination/4(VTQD_LimpHomeAct_flg)
  [VTQR_EVDriveMode_enum] -> Front wheel rate limit determination/5(VTQR_EVDriveMode_enum)
  [VDHP_ActAPSPosn_pct] -> Front wheel rate limit determination/6(VDHP_ActAPSPosn_pct)
  [VTQR_FEDUWhlTqReqSmoothDelay_Nm] -> Front wheel rate limit determination/7(VTQR_FEDUWhlTqReqSmoothDelay_Nm)
  [VTQD_EVDriveModeValid_flg] -> Front wheel rate limit determination/8(VTQD_EVDriveModeValid_flg)
  [VTQD_LimpHomeAct_flg] -> Rear wheel rate limit determination/4(VTQD_LimpHomeAct_flg)
  [VTQR_EVDriveMode_enum] -> Rear wheel rate limit determination/5(VTQR_EVDriveMode_enum)
  [VDHP_ActAPSPosn_pct] -> Rear wheel rate limit determination/6(VDHP_ActAPSPosn_pct)
  [VTQR_REDUWhlTqReqSmoothDelay_Nm] -> Rear wheel rate limit determination/7(VTQR_REDUWhlTqReqSmoothDelay_Nm)
  [VTQD_EVDriveModeValid_flg] -> Rear wheel rate limit determination/8(VTQD_EVDriveModeValid_flg)
  [VTQD_EVDriveModeValid_flg] -> Rear First order filter input tau map and determination/9(VTQD_EVDriveModeValid_flg)
  [VTQD_EVDriveModeValid_flg] -> Front First order filter input tau map and determination/9(VTQD_EVDriveModeValid_flg)
  [VTQD_TqTargetShaftSpd_rpm] -> Front Torque zero point transfer boundary map/1(VTQD_TqTargetShaftSpd_rpm)
  [VTQR_EVDriveMode_enum] -> Front Torque zero point transfer boundary map/2(VTQR_EVDriveMode_enum)
  Front Torque zero point transfer boundary map/1(VTQR_FrTqZeroTransUpBound_Nm) -> [VTQR_FrTqZeroTransUpBound_Nm]
  Front Torque zero point transfer boundary map/2(VTQR_FrTqZeroTransLowBound_Nm) -> [VTQR_FrTqZeroTransLowBound_Nm]
  [VTQD_TqTargetShaftSpd_rpm] -> Rear Torque zero point transfer boundary map/1(VTQD_TqTargetShaftSpd_rpm)
  [VTQR_EVDriveMode_enum] -> Rear Torque zero point transfer boundary map/2(VTQR_EVDriveMode_enum)
  Rear Torque zero point transfer boundary map/1(VTQR_RrTqZeroTransUpBound_Nm) -> [VTQR_RrTqZeroTransUpBound_Nm]
  Rear Torque zero point transfer boundary map/2(VTQR_RrTqZeroTransLowBound_Nm) -> [VTQR_RrTqZeroTransLowBound_Nm]
  [VTQD_RegenMode_enum] -> Front First order filter input tau map and determination/10(VTQD_RegenMode_enum)
  VTQD_RegenMode_enum/1 -> [VTQD_RegenMode_enum]
  [VTQD_RegenMode_enum] -> Front wheel rate limit determination/9(VTQD_RegenMode_enum)
  [VTQD_RegenMode_enum] -> Rear First order filter input tau map and determination/10(VTQD_RegenMode_enum)
  [VTQD_RegenMode_enum] -> Rear wheel rate limit determination/9(VTQD_RegenMode_enum)
  VVMC_ACCPedalOvrd_flg/1 -> [VVMC_ACCPedalOvrd_flg]
  VVMC_CCPedalOvrd_flg/1 -> [VVMC_CCPedalOvrd_flg]
  RegenLV_inc5/1 -> Equal/2
  Equal/1 -> Switch/2
  RegenLV_inc6/1 -> Switch/1
  Switch/1 -> [VTQR_EVDriveMode_enum]  "VTQR_EVDriveMode_enum"
  [VTQD_GearActualPosn_enum] -> Equal/1
  VTQD_GearActualPosn_enum/1 -> [VTQD_GearActualPosn_enum]
  [VVMC_ACCPedalOvrd_flg] -> Front First order filter input tau map and determination/11(VVMC_ACCPedalOvrd_flg)
  [VVMC_CCPedalOvrd_flg] -> Front First order filter input tau map and determination/12(VVMC_CCPedalOvrd_flg)
  [VVMC_ACCPedalOvrd_flg] -> Front wheel rate limit determination/10(VVMC_ACCPedalOvrd_flg)
  [VVMC_CCPedalOvrd_flg] -> Front wheel rate limit determination/11(VVMC_CCPedalOvrd_flg)
  [VVMC_ACCPedalOvrd_flg] -> Rear First order filter input tau map and determination/11(VVMC_ACCPedalOvrd_flg)
  [VVMC_CCPedalOvrd_flg] -> Rear First order filter input tau map and determination/12(VVMC_CCPedalOvrd_flg)
  [VVMC_ACCPedalOvrd_flg] -> Rear wheel rate limit determination/10(VVMC_ACCPedalOvrd_flg)
  [VVMC_CCPedalOvrd_flg] -> Rear wheel rate limit determination/11(VVMC_CCPedalOvrd_flg)
  VTQD_TqTargetShaftSpd_rpm/1 -> [VTQD_TqTargetShaftSpd_rpm]
  VTQD_PreLoadHold_flg/1 -> [VTQD_PreLoadHold_flg]
  VTQD_PreLoadPreEn_flg/1 -> [VTQD_PreLoadPreEn_flg]
  [VTQD_PreLoadHold_flg] -> Rear First order filter input tau map and determination/13(VTQD_PreLoadHold_flg)
  [VTQD_PreLoadHold_flg] -> Front First order filter input tau map and determination/13(VTQD_PreLoadHold_flg)
  VTQR_NoABSFEDUWhlTqReq_Nm/1 -> [VTQR_NoABSFEDUWhlTqReq_Nm]
  VTQR_NoABSREDUWhlTqReq_Nm/1 -> [VTQR_NoABSREDUWhlTqReq_Nm]
  VTQD_CreepPrLoadEnable_flg/1 -> [VTQD_CreepPrLoadEnable_flg]
  VVMC_ADASActive_flg/1 -> [VVMC_ADASActive_flg]
  [VTQD_CreepPrLoadEnable_flg] -> Front First order filter input tau map and determination/15(VTQD_CreepPrLoadEnable_flg)
  [VTQD_CreepPrLoadEnable_flg] -> Rear First order filter input tau map and determination/15(VTQD_CreepPrLoadEnable_flg)
  [VTQD_CreepPrLoadEnable_flg] -> Front wheel rate limit determination/12(VTQD_CreepPrLoadEnable_flg)
  [VTQD_RDCActive_enum] -> Front wheel rate limit determination/14(VTQD_RDCActive_enum)
  [VTQD_PreLoadPreEn_flg] -> Front wheel rate limit determination/15(VTQD_PreLoadPreEn_flg)
  VTQD_RDCActive_enum/1 -> [VTQD_RDCActive_enum]
  [VTQD_PreLoadPreEn_flg] -> Rear wheel rate limit determination/15(VTQD_PreLoadPreEn_flg)
  [VTQD_CreepPrLoadEnable_flg] -> Rear wheel rate limit determination/12(VTQD_CreepPrLoadEnable_flg)
  [VTQD_RDCActive_enum] -> Rear wheel rate limit determination/14(VTQD_RDCActive_enum)
  Ground1/1 -> [VINP_SCPSystemMode_enum]
  [VTQD_RDCActive_enum] -> Front First order filter input tau map and determination/16(VTQD_RDCActive_enum)
  [VTQR_NoABSFEDUWhlTqReq_Nm] -> Front First order filter input tau map and determination/17(VTQR_NoABSFEDUWhlTqReq_Nm)
  [VTQR_RampFEDUWhlTqReq_Nm] -> Front First order filter input tau map and determination/18(VTQR_RampFEDUWhlTqReq_Nm)
  [VTQR_NoABSFEDUWhlTqReq_Nm] -> Front wheel rate limit determination/16(VTQR_NoABSFEDUWhlTqReq_Nm)
  [VTQR_RampFEDUWhlTqReq_Nm] -> Front wheel rate limit determination/17(VTQR_RampFEDUWhlTqReq_Nm)
  [VTQD_RDCActive_enum] -> Rear First order filter input tau map and determination/16(VTQD_RDCActive_enum)
  [VTQR_NoABSREDUWhlTqReq_Nm] -> Rear First order filter input tau map and determination/17(VTQR_NoABSREDUWhlTqReq_Nm)
  [VTQR_RampREDUWhlTqReq_Nm] -> Rear First order filter input tau map and determination/18(VTQR_RampREDUWhlTqReq_Nm)
  [VTQR_NoABSREDUWhlTqReq_Nm] -> Rear wheel rate limit determination/16(VTQR_NoABSREDUWhlTqReq_Nm)
  [VTQR_RampREDUWhlTqReq_Nm] -> Rear wheel rate limit determination/17(VTQR_RampREDUWhlTqReq_Nm)
  [VTQR_FrFirstOrderInpTq_Nm] -> Front First order filter input tau map and determination/19(VTQR_FrFirstOrderInpTq_Nm)
  [VTQR_FrFirstOrderInpTq_Nm] -> Front wheel rate limit determination/18(VTQR_FrFirstOrderInpTq_Nm)
  [VTQR_RrFirstOrderInpTq_Nm] -> Rear First order filter input tau map and determination/19(VTQR_RrFirstOrderInpTq_Nm)
  [VTQR_RrFirstOrderInpTq_Nm] -> Rear wheel rate limit determination/18(VTQR_RrFirstOrderInpTq_Nm)
  [VTQR_ActREDUTrqUpLim_Nm] -> Limit2/2
  [VTQR_ActREDUTrqLowLim_Nm] -> Limit2/3
  VVMC_ActMaxSlideRate_pct/1 -> [VVMC_ActMaxSlideRate_pct]
  VTQD_RegenTqLimitEn_flg/1 -> [VTQD_RegenTqLimitEn_flg]
  VTQD_PedAccTqEn_flg/1 -> [VTQD_PedAccTqEn_flg]
  [VVMC_ActMaxSlideRate_pct] -> Front First order filter input tau map and determination/14(VVMC_ActMaxSlideRate_pct)
  [VVMC_ActMaxSlideRate_pct] -> Front wheel rate limit determination/19(VVMC_ActMaxSlideRate_pct)
  [VTQD_PedAccTqEn_flg] -> Front wheel rate limit determination/20(VTQD_PedAccTqEn_flg)
  [VTQD_RegenTqLimitEn_flg] -> Front wheel rate limit determination/13(VTQD_RegenTqLimitEn_flg)
  [VTQD_PedAccTqEn_flg] -> Rear wheel rate limit determination/20(VTQD_PedAccTqEn_flg)
  [VVMC_ActMaxSlideRate_pct] -> Rear wheel rate limit determination/19(VVMC_ActMaxSlideRate_pct)
  [VVMC_ActMaxSlideRate_pct] -> Rear First order filter input tau map and determination/14(VVMC_ActMaxSlideRate_pct)
  [VTQD_PedAccTqEn_flg] -> Rear First order filter input tau map and determination/20(VTQD_PedAccTqEn_flg)
  Constant5/1 -> Relational Operator4/2
  Relational Operator4/1 -> AND/1
  Equal2/1 -> AND/4
  [VTQR_EVDriveMode_enum] -> Equal1/1
  Equal1/1 -> AND/3
  [VDHP_ActAPSPosn_pct] -> Relational Operator4/1
  [VINP_VehSpeed_kph] -> Relational Operator6/1
  Relational Operator6/1 -> AND/2
  AND/1 -> [VTQR_LaunchEn_flg]  "VTQR_LaunchEn_flg"
  [VTQD_RegenMode_enum] -> Equal2/1
  Constant6/1 -> Relational Operator6/2
  Constant2/1 -> Equal2/2
  Constant4/1 -> Equal1/2
  [VTQD_PedAccTqEn_flg] -> Front First order filter input tau map and determination/20(VTQD_PedAccTqEn_flg)
  [VTQD_RegenTqLimitEn_flg] -> Rear wheel rate limit determination/13(VTQD_RegenTqLimitEn_flg)
  [VTQR_RampFEDUWhlTqReq_Nm] -> VTQR_RampFEDUWhlTqReq_Nm/1  "VTQR_RampFEDUWhlTqReq_Nm"
  [VTQR_RampREDUWhlTqReq_Nm] -> VTQR_RampREDUWhlTqReq_Nm/1  "VTQR_RampREDUWhlTqReq_Nm"
  [VTQR_FrGearChange_flg] -> Front wheel first order filter input torque command determination/6(VTQR_FrGearChange_flg)
  [VTQR_FrFirstOrderOutTqDelay_Nm] -> Front wheel first order filter input torque command determination/5(VTQR_FrFirstOrderOutTqDelay_Nm)
  [VTQR_FrTqZeroTrans_enum] -> Front wheel first order filter input torque command determination/1(VTQR_FrTqZeroTrans_enum)
  [VTQD_AfterAvailableTqDemFr_Nm] -> Front wheel first order filter input torque command determination/4(VTQD_AfterAvailableTqDemFr_Nm)
  [VTQR_FrTqZeroTransLowBound_Nm] -> Front wheel first order filter input torque command determination/3(VTQR_FrTqZeroTransLowBound_Nm)
  [VTQR_FrTqZeroTransUpBound_Nm] -> Front wheel first order filter input torque command determination/2(VTQR_FrTqZeroTransUpBound_Nm)
  [VTQR_RrGearChange_flg] -> Rear wheel first order filter input torque command determination/6(VTQR_RrGearChange_flg)
  [VTQR_RrTqZeroTransUpBound_Nm] -> Rear wheel first order filter input torque command determination/2(VTQR_RrTqZeroTransUpBound_Nm)
  [VTQD_AfterAvailableTqDemRr_Nm] -> Rear wheel first order filter input torque command determination/4(VTQD_AfterAvailableTqDemRr_Nm)
  [VTQR_RrTqZeroTransLowBound_Nm] -> Rear wheel first order filter input torque command determination/3(VTQR_RrTqZeroTransLowBound_Nm)
  [VTQR_RrFirstOrderOutTqDelay_Nm] -> Rear wheel first order filter input torque command determination/5(VTQR_RrFirstOrderOutTqDelay_Nm)
  [VTQR_RrTqZeroTrans_enum] -> Rear wheel first order filter input torque command determination/1(VTQR_RrTqZeroTrans_enum)
  VTQR_RrGearChange_flg/1 -> [VTQR_RrGearChange_flg]
  VTQR_FrGearChange_flg/1 -> [VTQR_FrGearChange_flg]
  [VINP_SCPSystemMode_enum] -> Terminator2/1
  [VTQD_PreLoadPreEn_flg] -> Front First order filter input tau map and determination/21(VTQD_PreLoadPreEn_flg)
  [VTQD_PreLoadPreEn_flg] -> Rear First order filter input tau map and determination/21(VTQD_PreLoadPreEn_flg)
  RegenLV_inc1/1 -> Equal3/2
  Equal3/1 -> Switch1/2
  [VTQD_GearActualPosn_enum] -> Equal3/1
  Constant3/1 -> Switch1/1
  Constant7/1 -> Switch1/3
  Switch1/1 -> VTQR_RampTqCMDGain_c/1, [VTQR_RampTqCMDGain_c]  "VTQR_RampTqCMDGain_c"
  [VTQR_RampTqCMDGain_c] -> Front wheel first order filter input torque command determination/7(VTQR_RampTqCMDGain_c)
  [VTQR_RampTqCMDGain_c] -> Rear wheel first order filter input torque command determination/7(VTQR_RampTqCMDGain_c)
  VVMC_MSAWhlTqActive_flg/1 -> [VVMC_MSAWhlTqActive_flg]
  [VVMC_MSAWhlTqActive_flg] -> Front First order filter input tau map and determination/22(VVMC_MSAWhlTqActive_flg)
  [VVMC_MSAWhlTqActive_flg] -> Front wheel rate limit determination/21(VVMC_MSAWhlTqActive_flg)
  [VVMC_MSAWhlTqActive_flg] -> Rear First order filter input tau map and determination/22(VVMC_MSAWhlTqActive_flg)
  [VVMC_MSAWhlTqActive_flg] -> Rear wheel rate limit determination/21(VVMC_MSAWhlTqActive_flg)
  [task_time_s] -> Front torque ramp limtation and determination/7(task_time_s)
  [VTQR_REDUWhlTqReqSmoothDelay_Nm] -> Front torque ramp limtation and determination/3(VTQR_REDUWhlTqReqSmoothDelay_Nm)
  [VINP_RFRawWhlSpeed_kph] -> Front torque ramp limtation and determination/6(VINP_RFRawWhlSpeed_kph)
  [VTQD_AfterAvailableTqDemFr_Nm] -> Front torque ramp limtation and determination/1(VTQD_AfterAvailableTqDemFr_Nm)
  Front torque ramp limtation and determination/2(VTQR_ActFEDUTrqLowLim_Nm) -> [VTQR_ActFEDUTrqLowLim_Nm]
  [VPMM_DriveTrainSelect_enum] -> Front torque ramp limtation and determination/4(VPMM_DriveTrainSelect_enum)
  [VTQD_AfterAvailableTqDemRr_Nm] -> Front torque ramp limtation and determination/2(VTQD_AfterAvailableTqDemRr_Nm)
  Front torque ramp limtation and determination/1(VTQR_ActFEDUTrqUpLim_Nm) -> [VTQR_ActFEDUTrqUpLim_Nm]
  [VINP_LFRawWhlSpeed_kph] -> Front torque ramp limtation and determination/5(VINP_LFRawWhlSpeed_kph)
  [task_time_s] -> Rear torque ramp limtation and determination/7(task_time_s)
  [VINP_LRRawWhlSpeed_kph] -> Rear torque ramp limtation and determination/5(VINP_LRRawWhlSpeed_kph)
  [VINP_RRRawWhlSpeed_kph] -> Rear torque ramp limtation and determination/6(VINP_RRRawWhlSpeed_kph)
  [VPMM_DriveTrainSelect_enum] -> Rear torque ramp limtation and determination/4(VPMM_DriveTrainSelect_enum)
  [VTQR_FEDUWhlTqReqSmoothDelay_Nm] -> Rear torque ramp limtation and determination/3(VTQR_FEDUWhlTqReqSmoothDelay_Nm)
  [VTQD_AfterAvailableTqDemFr_Nm] -> Rear torque ramp limtation and determination/1(VTQD_AfterAvailableTqDemFr_Nm)
  Rear torque ramp limtation and determination/2(VTQR_ActREDUTrqLowLim_Nm) -> [VTQR_ActREDUTrqLowLim_Nm]
  [VTQD_AfterAvailableTqDemRr_Nm] -> Rear torque ramp limtation and determination/2(VTQD_AfterAvailableTqDemRr_Nm)
  Rear torque ramp limtation and determination/1(VTQR_ActREDUTrqUpLim_Nm) -> [VTQR_ActREDUTrqUpLim_Nm]
  VINP_LFRawWhlSpeed_kph/1 -> [VINP_LFRawWhlSpeed_kph]
  VINP_LRRawWhlSpeed_kph/1 -> [VINP_LRRawWhlSpeed_kph]
  VINP_RRRawWhlSpeed_kph/1 -> [VINP_RRRawWhlSpeed_kph]
  VINP_RFRawWhlSpeed_kph/1 -> [VINP_RFRawWhlSpeed_kph]
  VINP_ACCVehHoldReq_flg/1 -> [VINP_ACCVehHoldReq_flg]
  VINP_GRADE_Deg/1 -> [VINP_GRADE_Deg]
  [VINP_ACCVehHoldReq_flg] -> Rear wheel rate limit determination/22(VINP_ACCVehHoldReq_flg)
  [VINP_GRADE_Deg] -> Rear wheel rate limit determination/23(VINP_GRADE_Deg)
  VTQD_VehActSpd_kph/1 -> [VTQD_VehActSpd_kph]
  [VTQD_VehActSpd_kph] -> Rear wheel rate limit determination/24(VTQD_VehActSpd_kph)
  [VVMC_ADASActive_flg] -> Rear wheel rate limit determination/25(VVMC_ADASActive_flg)
  [VPMM_DriveTrainSelect_enum] -> Rear wheel rate limit determination/26(VPMM_DriveTrainSelect_enum)
  [VTQD_PreLoadPreEn_flg] -> "Rear Torque zero point transfer status determination "/6(VTQD_PreLoadPreEn_flg)
  [VVMC_ACCPedalOvrd_flg] -> "Rear Torque zero point transfer status determination "/8(VVMC_ACCPedalOvrd_flg)
  [VINP_VehSpeed_kph] -> "Rear Torque zero point transfer status determination "/12(VINP_VehSpeed_kph)
  [VVMC_EstSlope_Deg] -> "Rear Torque zero point transfer status determination "/9(VVMC_EstSlope_Deg)
  [VTQR_LaunchEn_flg] -> "Rear Torque zero point transfer status determination "/7(VTQR_LaunchEn_flg)
  "Rear Torque zero point transfer status determination "/1(VTQR_RrTqZeroTrans_enum) -> [VTQR_RrTqZeroTrans_enum]
  [VTQD_CreepPrLoadEnable_flg] -> "Rear Torque zero point transfer status determination "/4(VTQD_CreepPrLoadEnable_flg)
  [VTQR_RrTqZeroTransUpBound_Nm] -> "Rear Torque zero point transfer status determination "/2(VTQR_RrTqZeroTransUpBound_Nm)
  [VTQD_AfterAvailableTqDemRr_Nm] -> "Rear Torque zero point transfer status determination "/11(VTQD_AfterAvailableTqDemRr_Nm)
  [VTQD_RegenMode_enum] -> "Rear Torque zero point transfer status determination "/10(VTQD_RegenMode_enum)
  [VTQR_RrTqZeroTransLowBound_Nm] -> "Rear Torque zero point transfer status determination "/3(VTQR_RrTqZeroTransLowBound_Nm)
  [VTQR_REDUWhlTqReqSmoothDelay_Nm] -> "Rear Torque zero point transfer status determination "/1(VTQR_REDUWhlTqReqSmoothDelay_Nm)
  [VVMC_ADASActive_flg] -> "Rear Torque zero point transfer status determination "/5(VVMC_ADASActive_flg)
  VVMC_EstSlope_Deg/1 -> [VVMC_EstSlope_Deg]
  [VTQD_CreepPrLoadEnable_flg] -> "Front Torque zero point transfer status determination "/4(VTQD_CreepPrLoadEnable_flg)
  [VTQR_FrTqZeroTransLowBound_Nm] -> "Front Torque zero point transfer status determination "/3(VTQR_FrTqZeroTransLowBound_Nm)
  [VTQD_PreLoadPreEn_flg] -> "Front Torque zero point transfer status determination "/6(VTQD_PreLoadPreEn_flg)
  [VTQR_LaunchEn_flg] -> "Front Torque zero point transfer status determination "/7(VTQR_LaunchEn_flg)
  [VVMC_EstSlope_Deg] -> "Front Torque zero point transfer status determination "/9(VVMC_EstSlope_Deg)
  [VTQD_AfterAvailableTqDemFr_Nm] -> "Front Torque zero point transfer status determination "/11(VTQD_AfterAvailableTqDemFr_Nm)
  "Front Torque zero point transfer status determination "/1(VTQR_FrTqZeroTrans_enum) -> [VTQR_FrTqZeroTrans_enum]
  [VTQR_FrTqZeroTransUpBound_Nm] -> "Front Torque zero point transfer status determination "/2(VTQR_FrTqZeroTransUpBound_Nm)
  [VVMC_ADASActive_flg] -> "Front Torque zero point transfer status determination "/5(VVMC_ADASActive_flg)
  [VVMC_ACCPedalOvrd_flg] -> "Front Torque zero point transfer status determination "/8(VVMC_ACCPedalOvrd_flg)
  [VTQD_RegenMode_enum] -> "Front Torque zero point transfer status determination "/10(VTQD_RegenMode_enum)
  [VINP_VehSpeed_kph] -> "Front Torque zero point transfer status determination "/12(VINP_VehSpeed_kph)
  [VTQR_FEDUWhlTqReqSmoothDelay_Nm] -> "Front Torque zero point transfer status determination "/1(VTQR_FEDUWhlTqReqSmoothDelay_Nm)
  [VINP_RrPTCSActive_flg] -> Rear First order filter input tau map and determination/23(VINP_RrPTCSActive_flg)
  [VINP_IVISnowModeCmd_flg] -> Rear First order filter input tau map and determination/24(VINP_IVISnowModeCmd_flg)
  [VINP_FrPTCSActive_flg] -> Front First order filter input tau map and determination/23(VINP_FrPTCSActive_flg)
  VINP_FrPTCSActive_flg/1 -> [VINP_FrPTCSActive_flg]
  VINP_RrPTCSActive_flg/1 -> [VINP_RrPTCSActive_flg]
  VINP_IVISnowModeCmd_flg/1 -> [VINP_IVISnowModeCmd_flg]
  [VINP_IVISnowModeCmd_flg] -> Front First order filter input tau map and determination/24(VINP_IVISnowModeCmd_flg)
  [VTQD_EVDriveMode_enum] -> Switch2/3
  [VINP_IVISnowModeCmd_flg] -> Switch2/2
  RegenLV_inc2/1 -> Switch2/1
  Switch2/1 -> Switch/3
  [VINP_RrPTCSActive_flg] -> Rear wheel rate limit determination/27(VINP_RrPTCSActive_flg)
  [VINP_IVISnowModeCmd_flg] -> Rear wheel rate limit determination/28(VINP_IVISnowModeCmd_flg)
  [VINP_FrPTCSActive_flg] -> Front wheel rate limit determination/22(VINP_FrPTCSActive_flg)
  [VINP_IVISnowModeCmd_flg] -> Front wheel rate limit determination/23(VINP_IVISnowModeCmd_flg)
  VINP_VehicleType_enum/1 -> [VINP_VehicleType_enum]
  [VINP_VehicleType_enum] -> Front wheel rate limit determination/24(VINP_VehicleType_enum)
  [VINP_VehicleType_enum] -> Rear wheel rate limit determination/29(VINP_VehicleType_enum)
  [VINP_VehicleType_enum] -> Rear First order filter input tau map and determination/25(VINP_VehicleType_enum)
  [VINP_VehicleType_enum] -> Front First order filter input tau map and determination/25(VINP_VehicleType_enum)

== system tqr/TQR/Determine Torque Request/TorqueArbitrament/TorqueSmooth/FirstOrderFilter ==
  in : Inport
  Tc : Inport  Port=2
  Ts : Inport  Port=3
  Add : Sum
  Add2 : Sum  Inputs=+-
  Constant3 : Constant  OutDataTypeStr=single
  Constant4 : Constant  Value=0  OutDataTypeStr=single
  Constant5 : Constant  Value=0  OutDataTypeStr=single
  Constant6 : Constant  Value=eps  OutDataTypeStr=single
  Divide : Product  Inputs=*/
  MinMax{1..4} (4 alike) : MinMax  Function=max  Inputs=2
  Product : Product  RndMeth=Zero
  Product1 : Product  RndMeth=Zero
  Unit Delay : UnitDelay  SampleTime=-1  HasFrameUpgradeWarning=on
  out : Outport
  wires:
  Add/1 -> out/1, Unit Delay/1
  Divide/1 -> Product1/1, Add2/2
  Constant3/1 -> Add2/1
  Add2/1 -> Product/2
  Product/1 -> Add/1
  Unit Delay/1 -> Product/1
  in/1 -> Product1/2
  Product1/1 -> Add/2
  Tc/1 -> MinMax2/1
  Constant4/1 -> MinMax2/2
  Ts/1 -> MinMax3/1
  Constant5/1 -> MinMax3/2
  MinMax3/1 -> MinMax1/2
  MinMax2/1 -> Divide/1, MinMax1/1
  MinMax1/1 -> MinMax4/1
  Constant6/1 -> MinMax4/2
  MinMax4/1 -> Divide/2
